simulink model "Simulink_testing"  (R2023b)
settings: Solver=VariableStepAuto  StartTime=0.0  StopTime=10.0  RelTol=1e-3
libraries: dspsnks4 x1, simulink x1, audiosources x1
settings Model: Creator=nickl  LastModifiedBy=nickl

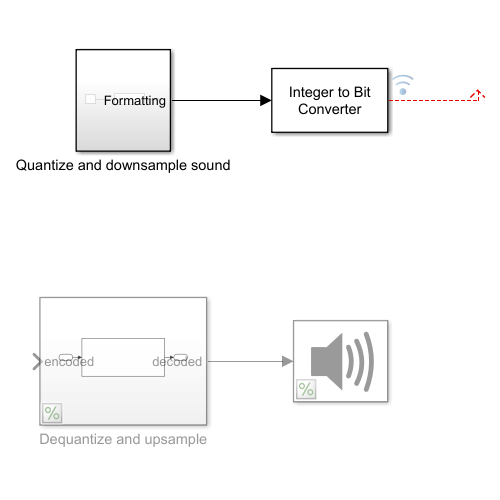
[thumbnail: Simulink's stored preview of the top-level diagram]
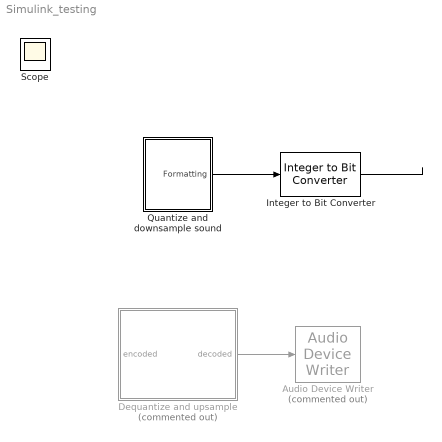
== system Simulink_testing ==
  Audio Device Writer : dspsnks4/Audio Device Writer  Commented=on  Driver=DirectSound  Device=Default  InheritSampleRate=on  SampleRate=44100  BitDepth=16-bit integer  BufferSize=4096  NumBuffers=10  DefaultOutputChannelMapping=on  OutputChannelMapping=1:2  OutputNumUnderrunSamples=off  DriverIdx=1  DeviceWarnFlag=''
  Dequantize and upsample : Subsystem  Commented=on
  Integer to Bit Converter : simulink/Logic and Bit Operations/Integer to Bit Converter  nbits=8  signedInputValues=Signed  bitOrder=MSB first  outDtype=Inherit via internal rule
      settings: LibrarySourceBlock=|
      | commutil2/Integer to Bit
      | Converter
  Quantize and downsample sound : Subsystem
  Scope : Scope
  wires:
  Quantize and downsample sound/1(Formatting) -> Integer to Bit Converter/1
  Dequantize and upsample/1(decoded) -> Audio Device Writer/1
  Integer to Bit Converter/1 -> ?

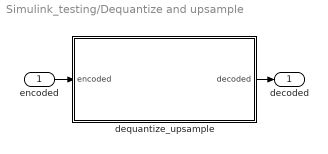
== system Simulink_testing/Dequantize and upsample ==
  encoded : Inport
  dequantize_upsample : MATLAB Function  TreatAsAtomicUnit=on
  decoded : Outport
  wires:
  encoded/1 -> dequantize_upsample/1(encoded)
  dequantize_upsample/1(decoded) -> decoded/1

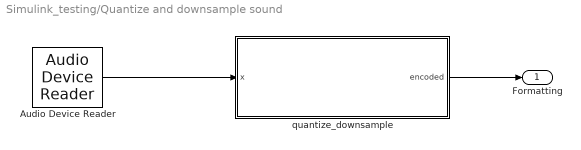
== system Simulink_testing/Quantize and downsample sound ==
  Audio Device Reader : audiosources/Audio Device Reader  Driver=DirectSound  Device=Microphone Array (AMD Audio Device)  SampleRate=44100  NumChannels=1  SamplesPerFrame=1024  BitDepth=16-bit integer  NumBuffers=10  DefaultInputChannelMapping=on  InputChannelMapping=1:2  OutputNumOverrunSamples=off  OutputDataType=double  DriverIdx=1  DeviceWarnFlag=''
  quantize_downsample : MATLAB Function  TreatAsAtomicUnit=on
  Formatting : Outport
  wires:
  quantize_downsample/1(encoded) -> Formatting/1
  Audio Device Reader/1 -> quantize_downsample/1(x)

== matlab function Simulink_testing/Dequantize and upsample/dequantize_upsample ==
  data: encoded input; decoded output size=[1024,1]
function decoded = dequantize_upsample(encoded)
    % Convert back to double in range [-1, 1]
    num_bits = 8;
    max_val = 2^(num_bits - 1) - 1;
    decoded = double(encoded) / max_val;

    % Upsample back to 44100 Hz
    fs_in = 8000;
    target_fs = 44100;
    
    % Check if encoded data is empty or has wrong size
    if isempty(decoded)
        error('Error: encoded input is empty.');
    end

    % Perform resampling
    decoded_resampled = resample(decoded, target_fs, fs_in);

    % Debugging: Display size of resampled output

    % Force exactly 1024 samples using interpolation
    decoded = decoded_resampled(1:1024);
    disp(decoded); 

end

== matlab function Simulink_testing/Quantize and downsample sound/quantize_downsample ==
  data: x input; encoded output
function encoded = quantize_downsample(x)
    if size(x,2) > 1
        x = mean(x,2); % Convert to mono
    end
    disp(x)
    % Define parameters
    num_bits = 8;
    target_fs = 8000;
    fs_in = 44100; % Set based on your input

    % Downsample from 44.1 kHz to 8 kHz
    x = resample(x, target_fs, fs_in);

    % Scale to integer range (quantization)
    max_val = 2^(num_bits - 1) - 1;
    x = round(x * max_val);
    
    % Convert to 8-bit integer
    encoded = int8(x);
    disp(size(encoded));
end
